simulink model "fuzzy_pid"  (Simulink 8.4)
settings: Solver=ode4  StartTime=0.0  StopTime=5  FixedStep=0.001  RelTol=1e-3
libraries: fuzblock x1, simulink x1
settings Model: Creator=Administrator  LastModifiedBy=Administrator
settings OptimizationCC: BlockReduction=off  BooleanDataType=off  ExpressionDepthLimit=128  InitFltsAndDblsToZero=on
settings DebuggingCC: SaveWithParameterizedLinksMsg=none  SignalResolutionControl=TryResolveAllWithWarning  MultiTaskDSMMsg=warning  MultiTaskCondExecSysMsg=none  StateNameClashWarn=none
settings RTWCC: IncludeERTFirstTime=on
settings GRTTargetCC: TargetFcnLib=ansi_tfl_tmw.mat

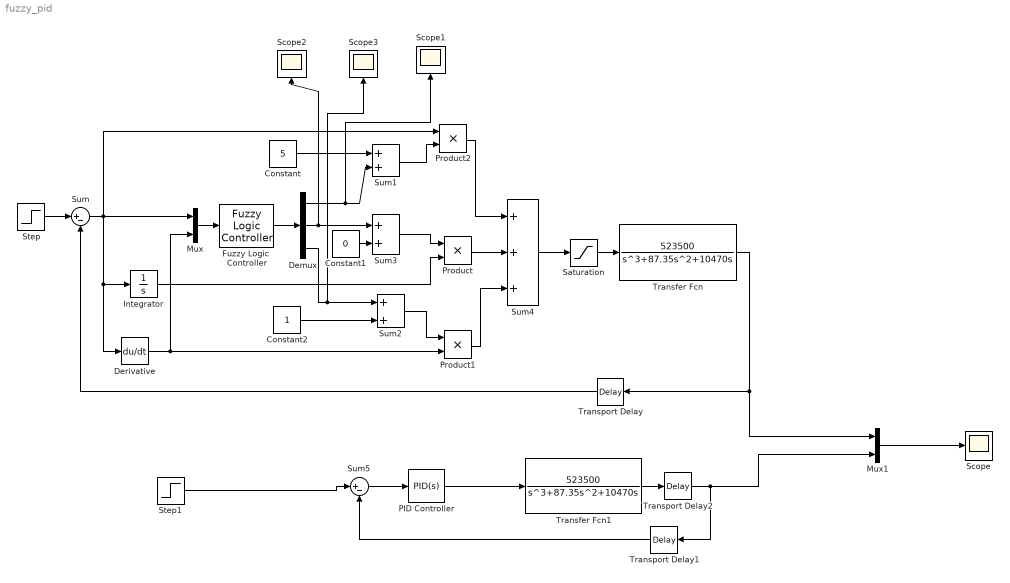
== system fuzzy_pid ==
  Constant : Constant  Value=5
  Constant1 : Constant  Value=0
  Constant2 : Constant
  Demux : Demux  Outputs=3
  Derivative : Derivative
  Fuzzy Logic  Controller : fuzblock/Fuzzy Logic  Controller  fis=fuzzy02
  Integrator : Integrator
  Mux : Mux  Inputs=2
  Mux1 : Mux  Inputs=2
  PID Controller : simulink/Continuous/PID Controller  Controller=PID  TimeDomain=Continuous-time  SampleTime=-1  IntegratorMethod=Forward Euler  FilterMethod=Forward Euler  Form=Parallel  P=0.714902143194451  I=0.198807443563222  D=-0.0085328033532702  N=31.6752409861176  InitialConditionSource=internal  InitialConditionForIntegrator=0  InitialConditionForFilter=0  ExternalReset=none  LimitOutput=off  UpperSaturationLimit=inf  LowerSaturationLimit=-inf  LinearizeAsGain=on  AntiWindupMode=none  Kb=1  TrackingMode=off  Kt=1  PParamMin=[]  PParamMax=[]  IParamMin=[]  IParamMax=[]  DParamMin=[]  DParamMax=[]  NParamMin=[]  NParamMax=[]  KbParamMin=[]  KbParamMax=[]  KtParamMin=[]  KtParamMax=[]  POutMin=[]  POutMax=[]  IOutMin=[]  IOutMax=[]  DOutMin=[]  DOutMax=[]  NOutMin=[]  NOutMax=[]  KbOutMin=[]  KbOutMax=[]  KtOutMin=[]  KtOutMax=[]  IntegratorOutMin=[]  IntegratorOutMax=[]  FilterOutMin=[]  FilterOutMax=[]  SumOutMin=[]  SumOutMax=[]  SumI1OutMin=[]  SumI1OutMax=[]  SumI2OutMin=[]  SumI2OutMax=[]  SumI3OutMin=[]  SumI3OutMax=[]  SumDOutMin=[]  SumDOutMax=[]  SaturationOutMin=[]  SaturationOutMax=[]  IntegratorContinuousStateAttributes=''  IntegratorStateMustResolveToSignalObject=off  IntegratorRTWStateStorageClass=Auto  FilterContinuousStateAttributes=''  FilterStateMustResolveToSignalObject=off  FilterRTWStateStorageClass=Auto  DifferentiatorICPrevScaledInput=0  DifferentiatorOutMin=[]  DifferentiatorOutMax=[]  UseFilter=on
  Product : Product  RndMeth=Zero
  Product1 : Product  RndMeth=Zero
  Product2 : Product  RndMeth=Zero
  Saturation : Saturate
  Scope{,1..3} (4 alike) : Scope
      Scope settings: TimeRange=2  YMin=0.7  YMax=1.3  MaxDataPoints=5000000
      Scope2 settings: YMin=1.4e-008  YMax=2.9e-008  SaveName=ScopeData2
      Scope3 settings: SaveName=ScopeData3
  Step : Step  Time=0  SampleTime=0
  Step1 : Step  Time=0  SampleTime=0
  Sum : Sum  Inputs=|+-
  Sum1 : Sum
  Sum2 : Sum
  Sum3 : Sum
  Sum4 : Sum  Inputs=+++
  Sum5 : Sum  Inputs=|+-
  Transfer Fcn : TransferFcn  Numerator=[523500]  Denominator=[1 87.35 10470 0]
  Transfer Fcn1 : TransferFcn  Numerator=[523500]  Denominator=[1 87.35 10470 0]
  Transport Delay : TransportDelay  DelayTime=0.01
  Transport Delay1 : TransportDelay  DelayTime=0.001
  Transport Delay2 : TransportDelay  DelayTime=0.001
  wires:
  Fuzzy Logic  Controller/1 -> Demux/1
  Sum/1 -> Mux/1, Product2/1, Derivative/1, Integrator/1
  Step/1 -> Sum/1
  Mux/1 -> Fuzzy Logic  Controller/1
  Transfer Fcn/1 -> Mux1/1, Transport Delay/1
  Derivative/1 -> Mux/2, Product1/2
  Demux/1 -> Sum1/2, Scope1/1
  Constant/1 -> Sum1/1
  Sum1/1 -> Product2/2
  Constant2/1 -> Sum2/2
  Sum2/1 -> Product1/1
  Constant1/1 -> Sum3/2
  Integrator/1 -> Product/2
  Sum3/1 -> Product/1
  Product2/1 -> Sum4/1
  Sum4/1 -> Saturation/1
  Demux/2 -> Sum3/1, Scope2/1
  Saturation/1 -> Transfer Fcn/1
  Demux/3 -> Sum2/1, Scope3/1
  Product/1 -> Sum4/2
  Product1/1 -> Sum4/3
  Step1/1 -> Sum5/1
  Sum5/1 -> PID Controller/1
  PID Controller/1 -> Transfer Fcn1/1
  Mux1/1 -> Scope/1
  Transfer Fcn1/1 -> Transport Delay2/1
  Transport Delay/1 -> Sum/2
  Transport Delay1/1 -> Sum5/2
  Transport Delay2/1 -> Transport Delay1/1, Mux1/2
